simulink model "simulacion"  (R2020a)
settings: Solver=VariableStepAuto  StartTime=0.0  StopTime=5.0  RelTol=1e-3
values from neighbouring files (symbols this model uses):
  beq = bm+(bl/r^2)    (= 1.5e-05)    [Parametros.m]
  Cts = 1.091    [Parametros.m]
  Jeq = Jm+(Jl/r^2)    (= 5.65099476805e-06)    [Parametros.m]
  lambdam = .01546    (= 0.01546)    [Parametros.m]
  Ld = 6.6e-3    (= 0.0066)    [Parametros.m]
  Lls = 0.8e-3    (= 0.0008)    [Parametros.m]
  Lq = 5.8e-3    (= 0.0058)    [Parametros.m]
  Pp = 3    [Parametros.m]
  r = 314.3008    [Parametros.m]
  Rs40 = 1.02    [Parametros.m]
  Rts = 55    [Parametros.m]
settings Model: Creator=tinsu  LastModifiedBy=tinsu

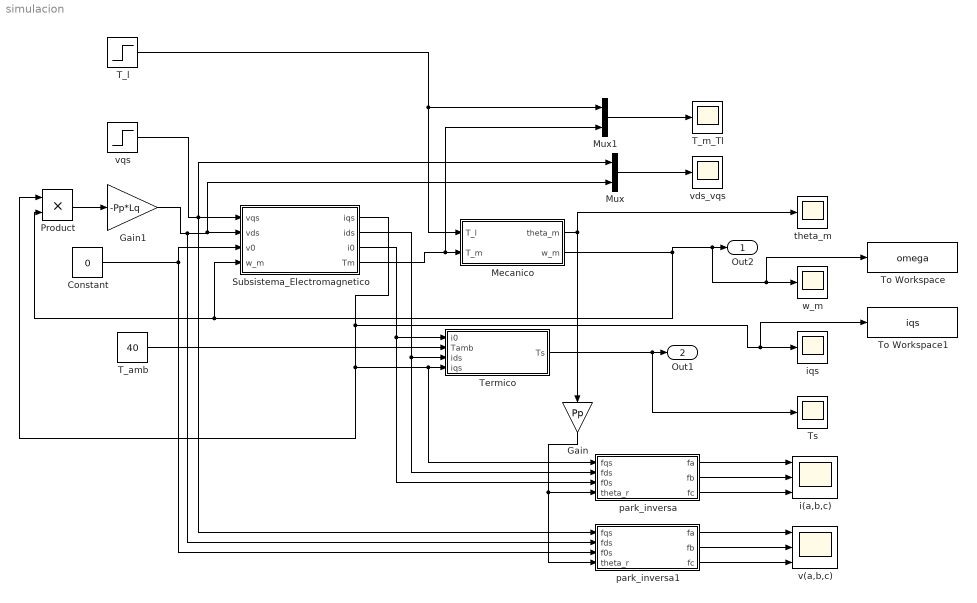
== system simulacion ==
  Constant : Constant  Value=0
  Gain : Gain  Gain=Pp
  Gain1 : Gain  Gain=-Pp*Lq
  Mecanico : Subsystem
  Mux : Mux  Inputs=2
  Mux1 : Mux  Inputs=2
  Product : Product
  Subsistema_Electromagnetico : Subsystem
  T_amb : Constant  Value=40
  T_l : Step  Time=0.3  After=1.57  SampleTime=0
  T_m_Tl : Scope
  Termico : Subsystem
  To Workspace : ToWorkspace  VariableName=omega  SampleTime=0.0001
  To Workspace1 : ToWorkspace  VariableName=iqs  SampleTime=0.0001
  Ts : Scope
  i(a,b,c) : Scope  NumInputPorts=3
  iqs : Scope
  park_inversa : Subsystem
  park_inversa1 : Subsystem
  theta_m : Scope
  v(a,b,c) : Scope  NumInputPorts=3
  vds_vqs : Scope
  vqs : Step  Time=0.1  After=19.596  SampleTime=0
  w_m : Scope
  Out2 : Outport
  Out1 : Outport  Port=2
  wires:
  Subsistema_Electromagnetico/4(Tm) -> Mux1/2, Mecanico/2(T_m)
  Subsistema_Electromagnetico/3(i0) -> park_inversa/3(f0s), Termico/1(i0)
  Subsistema_Electromagnetico/2(ids) -> Termico/3(ids), park_inversa/2(fds)
  Subsistema_Electromagnetico/1(iqs) -> To Workspace1/1, iqs/1, Product/1, park_inversa/1(fqs), Termico/4(iqs)
  Mecanico/2(w_m) -> To Workspace/1, w_m/1, Out2/1, Product/2, Subsistema_Electromagnetico/4(w_m)
  Constant/1 -> Subsistema_Electromagnetico/3(v0), park_inversa1/3(f0s)
  vqs/1 -> park_inversa1/1(fqs), Subsistema_Electromagnetico/1(vqs), Mux/1
  T_amb/1 -> Termico/2(Tamb)
  T_l/1 -> Mux1/1, Mecanico/1(T_l)
  Mecanico/1(theta_m) -> theta_m/1, Gain/1
  park_inversa/1(fa) -> i(a,b,c)/1
  park_inversa/2(fb) -> i(a,b,c)/2
  park_inversa/3(fc) -> i(a,b,c)/3
  park_inversa1/1(fa) -> v(a,b,c)/1
  park_inversa1/2(fb) -> v(a,b,c)/2
  park_inversa1/3(fc) -> v(a,b,c)/3
  Product/1 -> Gain1/1
  Gain1/1 -> park_inversa1/2(fds), Mux/2, Subsistema_Electromagnetico/2(vds)
  Termico/1(Ts) -> Ts/1, Out1/1
  Gain/1 -> park_inversa1/4(theta_r), park_inversa/4(theta_r)
  Mux/1 -> vds_vqs/1
  Mux1/1 -> T_m_Tl/1

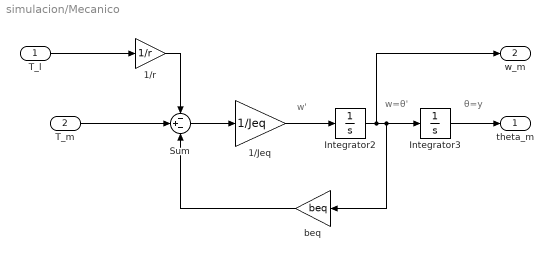
== system simulacion/Mecanico ==
  note: w=θ'
  note: θ=y
  note: w'
  T_l : Inport
  T_m : Inport  Port=2
  "1/Jeq " : Gain  Gain=1/Jeq
  "1/r " : Gain  Gain=1/r
  Integrator2 : Integrator
  Integrator3 : Integrator
  Sum : Sum  Inputs=-+-
  "beq " : Gain  Gain=beq
  theta_m : Outport
  w_m : Outport  Port=2
  wires:
  "1/r "/1 -> Sum/1
  "1/Jeq "/1 -> Integrator2/1
  Integrator3/1 -> theta_m/1
  Sum/1 -> "1/Jeq "/1
  "beq "/1 -> Sum/3
  Integrator2/1 -> Integrator3/1, "beq "/1, w_m/1
  T_m/1 -> Sum/2
  T_l/1 -> "1/r "/1

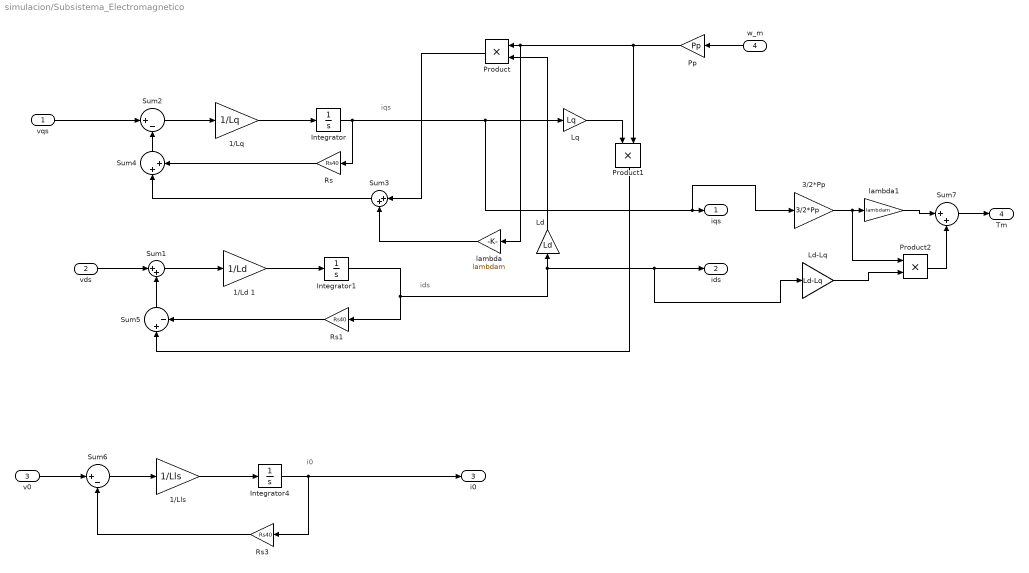
== system simulacion/Subsistema_Electromagnetico ==
  note: iqs
  note: i0
  note: ids
  vqs : Inport
  vds : Inport  Port=2
  v0 : Inport  Port=3
  w_m : Inport  Port=4
  1/Ld 1 : Gain  Gain=1/Ld
  1/Lls : Gain  Gain=1/Lls
  "1/Lq " : Gain  Gain=1/Lq
  3/2*Pp : Gain  Gain=3/2*Pp
  Integrator : Integrator
  Integrator1 : Integrator
  Integrator4 : Integrator
  Ld : Gain  Gain=Ld
  Ld-Lq : Gain  Gain=Ld-Lq
  "Lq " : Gain  Gain=Lq
  Pp : Gain  Gain=Pp
  Product : Product
  Product1 : Product
  Product2 : Product
  Rs : Gain  Gain=Rs40
  Rs1 : Gain  Gain=Rs40
  Rs3 : Gain  Gain=Rs40
  Sum{1,3..4,7} (4 alike) : Sum  Inputs=|++
  Sum2 : Sum  Inputs=|+-
  Sum5 : Sum  Inputs=|+-
  Sum6 : Sum  Inputs=|+-
  lambda : Gain  Gain=lambdam
  lambda1 : Gain  Gain=lambdam
  iqs : Outport
  ids : Outport  Port=2
  i0 : Outport  Port=3
  Tm : Outport  Port=4
  wires:
  Integrator4/1 -> i0/1, Rs3/1
  Sum6/1 -> 1/Lls/1
  Sum5/1 -> Sum1/2
  Rs/1 -> Sum4/2
  Sum4/1 -> Sum2/2
  "1/Lq "/1 -> Integrator/1
  Integrator1/1 -> Rs1/1, Ld-Lq/1, ids/1, Ld/1
  Integrator/1 -> Rs/1, 3/2*Pp/1, iqs/1, "Lq "/1
  Rs3/1 -> Sum6/2
  1/Lls/1 -> Integrator4/1
  Product/1 -> Sum3/1
  Pp/1 -> lambda/1, Product/1, Product1/2
  "Lq "/1 -> Product1/1
  Sum1/1 -> 1/Ld 1/1
  Product1/1 -> Sum5/1
  1/Ld 1/1 -> Integrator1/1
  Sum2/1 -> "1/Lq "/1
  v0/1 -> Sum6/1
  lambda/1 -> Sum3/2
  Ld/1 -> Product/2
  Rs1/1 -> Sum5/2
  vds/1 -> Sum1/1
  Sum3/1 -> Sum4/1
  vqs/1 -> Sum2/1
  w_m/1 -> Pp/1
  Ld-Lq/1 -> Product2/2
  lambda1/1 -> Sum7/1
  Product2/1 -> Sum7/2
  3/2*Pp/1 -> Product2/1, lambda1/1
  Sum7/1 -> Tm/1

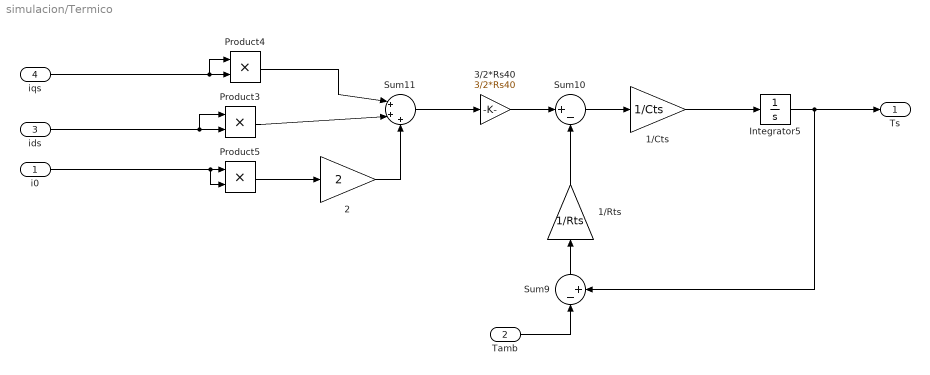
== system simulacion/Termico ==
  i0 : Inport
  Tamb : Inport  Port=2
  ids : Inport  Port=3
  iqs : Inport  Port=4
  1/Cts : Gain  Gain=1/Cts
  1/Rts : Gain  Gain=1/Rts
  "2 " : Gain  Gain=2
  "3/2*Rs40 " : Gain  Gain=3/2*Rs40
  Integrator5 : Integrator
  Product3 : Product
  Product4 : Product
  Product5 : Product
  Sum10 : Sum  Inputs=|+-
  Sum11 : Sum  Inputs=|+++
  Sum9 : Sum  Inputs=|-+
  Ts : Outport
  wires:
  "3/2*Rs40 "/1 -> Sum10/1
  1/Cts/1 -> Integrator5/1
  Sum10/1 -> 1/Cts/1
  Tamb/1 -> Sum9/1
  Integrator5/1 -> Ts/1, Sum9/2
  Product3/1 -> Sum11/2
  ids/1 -> Product3/1, Product3/2
  "2 "/1 -> Sum11/3
  Sum11/1 -> "3/2*Rs40 "/1
  Product5/1 -> "2 "/1
  i0/1 -> Product5/2, Product5/1
  1/Rts/1 -> Sum10/2
  Product4/1 -> Sum11/1
  Sum9/1 -> 1/Rts/1
  iqs/1 -> Product4/1, Product4/2

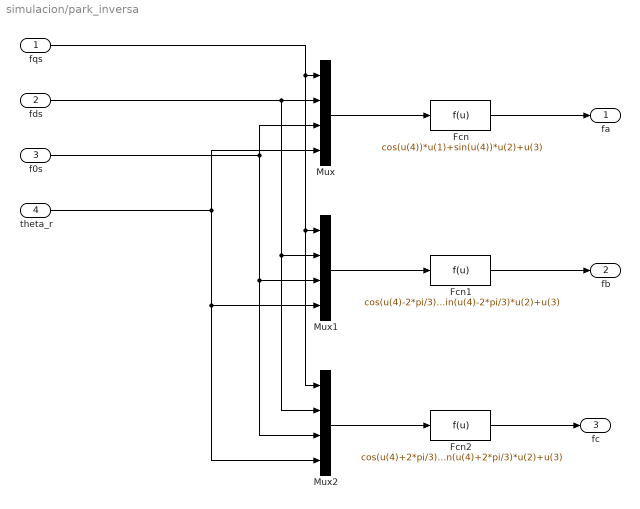
== system simulacion/park_inversa ==
  fqs : Inport
  fds : Inport  Port=2
  f0s : Inport  Port=3
  theta_r : Inport  Port=4
  Fcn : Fcn  Expr=cos(u(4))*u(1)+sin(u(4))*u(2)+u(3)
  Fcn1 : Fcn  Expr=cos(u(4)-2*pi/3)*u(1)+sin(u(4)-2*pi/3)*u(2)+u(3)
  Fcn2 : Fcn  Expr=cos(u(4)+2*pi/3)*u(1)+sin(u(4)+2*pi/3)*u(2)+u(3)
  Mux : Mux
  Mux1 : Mux
  Mux2 : Mux
  fa : Outport
  fb : Outport  Port=2
  fc : Outport  Port=3
  wires:
  f0s/1 -> Mux/3, Mux1/3, Mux2/3
  fds/1 -> Mux/2, Mux1/2, Mux2/2
  Fcn/1 -> fa/1
  Fcn2/1 -> fc/1
  theta_r/1 -> Mux/4, Mux1/4, Mux2/4
  Mux2/1 -> Fcn2/1
  Mux1/1 -> Fcn1/1
  Mux/1 -> Fcn/1
  Fcn1/1 -> fb/1
  fqs/1 -> Mux1/1, Mux2/1, Mux/1

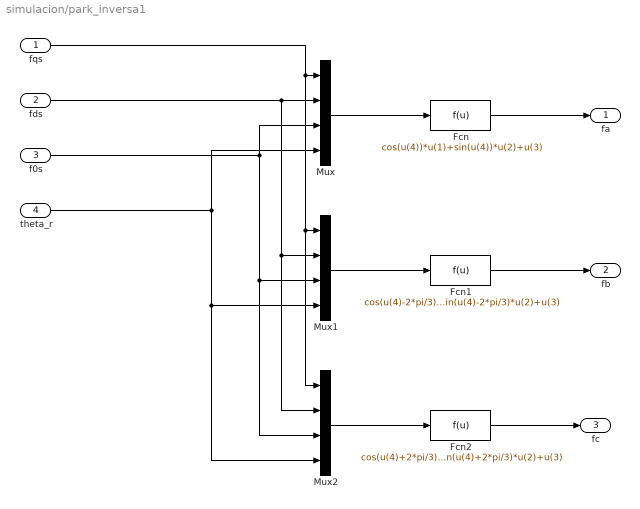
== system simulacion/park_inversa1 ==
  fqs : Inport
  fds : Inport  Port=2
  f0s : Inport  Port=3
  theta_r : Inport  Port=4
  Fcn : Fcn  Expr=cos(u(4))*u(1)+sin(u(4))*u(2)+u(3)
  Fcn1 : Fcn  Expr=cos(u(4)-2*pi/3)*u(1)+sin(u(4)-2*pi/3)*u(2)+u(3)
  Fcn2 : Fcn  Expr=cos(u(4)+2*pi/3)*u(1)+sin(u(4)+2*pi/3)*u(2)+u(3)
  Mux : Mux
  Mux1 : Mux
  Mux2 : Mux
  fa : Outport
  fb : Outport  Port=2
  fc : Outport  Port=3
  wires:
  f0s/1 -> Mux/3, Mux1/3, Mux2/3
  fds/1 -> Mux/2, Mux1/2, Mux2/2
  Fcn/1 -> fa/1
  Fcn2/1 -> fc/1
  theta_r/1 -> Mux/4, Mux1/4, Mux2/4
  Mux2/1 -> Fcn2/1
  Mux1/1 -> Fcn1/1
  Mux/1 -> Fcn/1
  Fcn1/1 -> fb/1
  fqs/1 -> Mux1/1, Mux2/1, Mux/1
